simulink model "matlab_q7"  (R2022b)
settings: Solver=VariableStepAuto  StartTime=0.0  StopTime=50.0  RelTol=1e-3
settings Model: Creator=NITRO  LastModifiedBy=NITRO

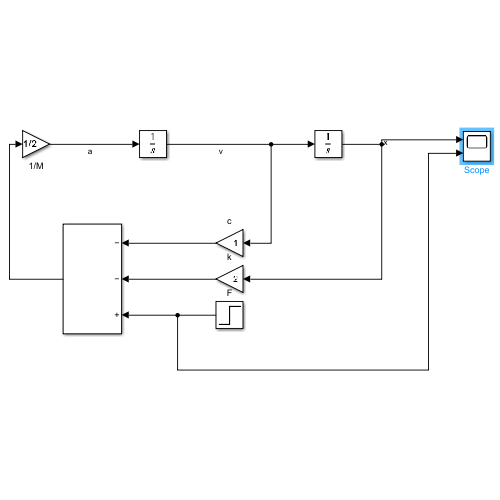
[thumbnail: Simulink's stored preview of the top-level diagram]
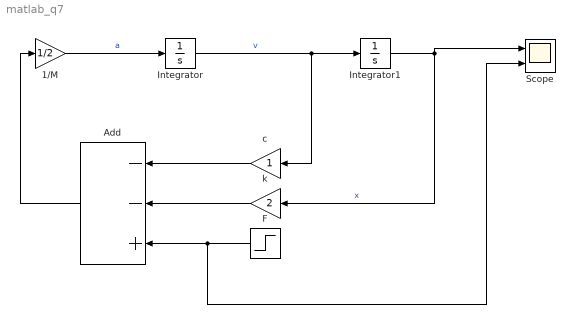
== system matlab_q7 ==
  1/M : Gain  Gain=1/2
  Add : Sum  Inputs=--+
  F : Step  Time=10  After=0.5  SampleTime=0
  Integrator : Integrator
  Integrator1 : Integrator  InitialCondition=0.4
  Scope : Scope  NumInputPorts=2
  c : Gain
  k : Gain  Gain=2
  wires:
  Integrator/1 -> c/1, Integrator1/1  "v"
  Integrator1/1 -> k/1, Scope/1  "x"
  c/1 -> Add/1
  k/1 -> Add/2
  Add/1 -> 1/M/1
  1/M/1 -> Integrator/1  "a"
  F/1 -> Scope/2, Add/3
